simulink model "OMSv1_2"  (Simulink 6.6)
settings: Solver=ode4  SolverMode=SingleTasking  StartTime=0.0  StopTime=5  FixedStep=0.001  MaxStep=0.001  RelTol=1e-3  AbsTol=1e-3
undefined symbols (not defined in the file): alexlaw, bs_onoff, bs_scale, bsfsacrit, bsfsvcrit, cnsgain, fs_onoff, fs_scale, fsdelaycalc, ltdrk, phasicgain, pmcgain, pmctau2, pmctau3, saccsw, spgain, tonicgain, tvrD, tvrN
(part 1 of 7)
CloseFcn:
  | ;slview('closediagram',bdroot);
settings Model: Creator=jacobs  LastModifiedBy=lfd  ExtModeAutoUpdateStatusClock=off
settings DataIOCC: LimitDataPoints=off  SaveOutput=off  SaveTime=off
settings OptimizationCC: BlockReduction=off  BooleanDataType=off
settings DebuggingCC: SignalResolutionControl=TryResolveAllWithWarning  SolverPrmCheckMsg=none  MultiTaskDSMMsg=warning  MultiTaskCondExecSysMsg=none  StrictBusMsg=None
settings HardwareCC: TargetUnknown=on
settings RTWCC: IncludeERTFirstTime=on
settings GRTTargetCC: ModelReferenceCompliant=off  MatFileLogging=off

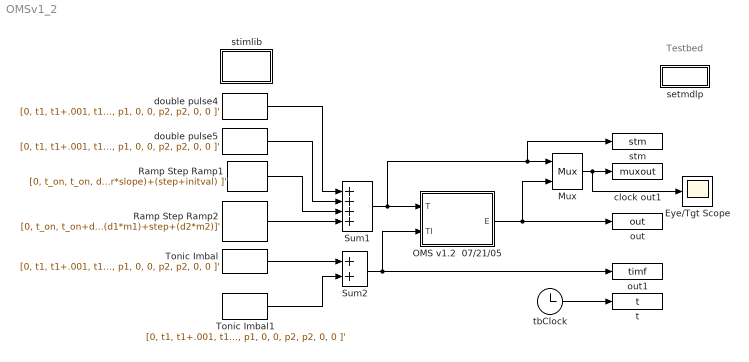
== system OMSv1_2 ==
  note: Testbed
  Eye/Tgt Scope : Scope
      settings: TickLabels=on  TimeRange=5  YMin=-5  YMax=32.5  DataFormat=Array
  Mux : Mux  Inputs=2
  OMS v1.2  07/21/05 : Subsystem
      mask init:
      | k=0.25;loadmdlp;prolong_buffersize=5120;
      mask Display: disp('OMS v1.2\nModel')
  Ramp Step Ramp1 : FromWorkspace  VariableName=[0, t_on, t_on, dur+t_on dur+t_on; initval, initval, initval+step, (dur*slope)+(step+initval), (dur*slope)+(step+initval) ]'  SampleTime=.001  mask{initval=0, t_on=1, step=0, dur=5, slope=0}
      mask prompts: initval "Initial value"; t_on "Time of step"; step "Size of step"; dur "Ramp duration"; slope "Ramp slope"
      mask help: Ramp Step Ramp
      mask Display: disp('Step\nRamp')
  Ramp Step Ramp2 : FromWorkspace  VariableName=[0, t_on, t_on+d1, t_on+d1, t_on+d1+d2, 10000; vi, vi, vi+(d1*m1), (vi+step)+(d1*m1), (vi+step)+(d1*m1)+(d2*m2), vi+(d1*m1)+step+(d2*m2)]'  SampleTime=.001  mask{vi=0, t_on=.25, d1=4, m1=0, step=0, d2=2, m2=0}
      mask prompts: vi "Initial value"; t_on "Time of first ramp"; d1 "First Ramp duration"; m1 "First Ramp slope"; step "Size of step"; d2 "Second Ramp duration"; m2 "Second Ramp slope"
      mask help: Ramp Step Ramp
      mask Display: disp('Ramp\nStep\nRamp')
  Sum1 : Sum  Inputs=++++  SaturateOnIntegerOverflow=on  InputSameDT=on
  Sum2 : Sum  SaturateOnIntegerOverflow=on  InputSameDT=on
  Tonic Imbal : FromWorkspace  VariableName=[0, t1, t1+.001, t1+d1, t1+d1+.001, t1+d1+.001+ipd, t1+d1+.001+ipd, t1+d1+.001+ipd+d2, t1+d1+.001+ipd+d2, 10000; 0, 0, p1, p1, 0, 0, p2, p2, 0, 0 ]'  SampleTime=.001  mask{@1=0, @2=0, @3=2, @4=0, @5=0, @6=3}
      mask prompts: @1 "Pulse 1 Magnitude"; @2 "Time of Pulse 1 Onset"; @3 "Pulse 1 Duration"; @4 "Interpulse Delay"; @5 "Pulse 2 Magnitude"; @6 "Pulse 2 Duration"
      mask help: Double Pulse
      mask init:
      | p1=@1; t1=@2; d1=@3; ipd=@4; p2=@5; d2=@6;
      mask Display: disp('Double\nPulse')
  Tonic Imbal1 : FromWorkspace  VariableName=[0, t1, t1+.001, t1+d1, t1+d1+.001, t1+d1+.001+ipd, t1+d1+.001+ipd, t1+d1+.001+ipd+d2, t1+d1+.001+ipd+d2, 10000; 0, 0, p1, p1, 0, 0, p2, p2, 0, 0 ]'  SampleTime=.001  mask{@1=0, @2=0, @3=3.5, @4=0, @5=0, @6=1.5}
      mask prompts: @1 "Pulse 1 Magnitude"; @2 "Time of Pulse 1 Onset"; @3 "Pulse 1 Duration"; @4 "Interpulse Delay"; @5 "Pulse 2 Magnitude"; @6 "Pulse 2 Duration"
      mask help: Double Pulse
      mask init:
      | p1=@1; t1=@2; d1=@3; ipd=@4; p2=@5; d2=@6;
      mask Display: disp('Double\nPulse')
  clock out1 : ToWorkspace  VariableName=muxout  SaveFormat=Array
      settings: MaxDataPoints=100000
  double pulse4 : FromWorkspace  VariableName=[0, t1, t1+.001, t1+d1, t1+d1+.001, t1+d1+.001+ipd, t1+d1+.001+ipd, t1+d1+.001+ipd+d2, t1+d1+.001+ipd+d2, 10000; 0, 0, p1, p1, 0, 0, p2, p2, 0, 0 ]'  SampleTime=.001  mask{@1=15, @2=2, @3=2, @4=0, @5=0, @6=5}
      mask prompts: @1 "Pulse 1 Magnitude"; @2 "Time of Pulse 1 Onset"; @3 "Pulse 1 Duration"; @4 "Interpulse Delay"; @5 "Pulse 2 Magnitude"; @6 "Pulse 2 Duration"
      mask help: Double Pulse
      mask init:
      | p1=@1; t1=@2; d1=@3; ipd=@4; p2=@5; d2=@6;
      mask Display: disp('Double\nPulse')
  double pulse5 : FromWorkspace  VariableName=[0, t1, t1+.001, t1+d1, t1+d1+.001, t1+d1+.001+ipd, t1+d1+.001+ipd, t1+d1+.001+ipd+d2, t1+d1+.001+ipd+d2, 10000; 0, 0, p1, p1, 0, 0, p2, p2, 0, 0 ]'  SampleTime=.001  mask{@1=0, @2=0, @3=1, @4=0, @5=0, @6=4.5}
      mask prompts: @1 "Pulse 1 Magnitude"; @2 "Time of Pulse 1 Onset"; @3 "Pulse 1 Duration"; @4 "Interpulse Delay"; @5 "Pulse 2 Magnitude"; @6 "Pulse 2 Duration"
      mask help: Double Pulse
      mask init:
      | p1=@1; t1=@2; d1=@3; ipd=@4; p2=@5; d2=@6;
      mask Display: disp('Double\nPulse')
  out : ToWorkspace  VariableName=out  SaveFormat=Array
      settings: MaxDataPoints=100000
  out1 : ToWorkspace  VariableName=timf  SaveFormat=Array
      settings: MaxDataPoints=100000
  setmdlp : Subsystem
      settings: OpenFcn=setmdlp
      mask Display: disp('setmdlp')
  stimlib : Subsystem
      settings: OpenFcn=stimlib
      mask Display: disp('Stimlib')
  stm : ToWorkspace  VariableName=stm  SaveFormat=Array
      settings: MaxDataPoints=100000
  t : ToWorkspace  VariableName=t  SaveFormat=Array
      mask init:
      | global t
      settings: MaxDataPoints=100000
  tbClock : Clock
      settings: Decimation=10
  wires:
  tbClock/1 -> t/1
  double pulse4/1 -> Sum1/1
  Sum1/1 -> OMS v1.2  07/21/05/1(T), stm/1, Mux/1
  OMS v1.2  07/21/05/1(E) -> out/1, Mux/2
  Mux/1 -> clock out1/1, Eye/Tgt Scope/1
  Tonic Imbal/1 -> Sum2/1
  Tonic Imbal1/1 -> Sum2/2
  Sum2/1 -> OMS v1.2  07/21/05/2(TI), out1/1
  double pulse5/1 -> Sum1/2
  Ramp Step Ramp1/1 -> Sum1/3
  Ramp Step Ramp2/1 -> Sum1/4

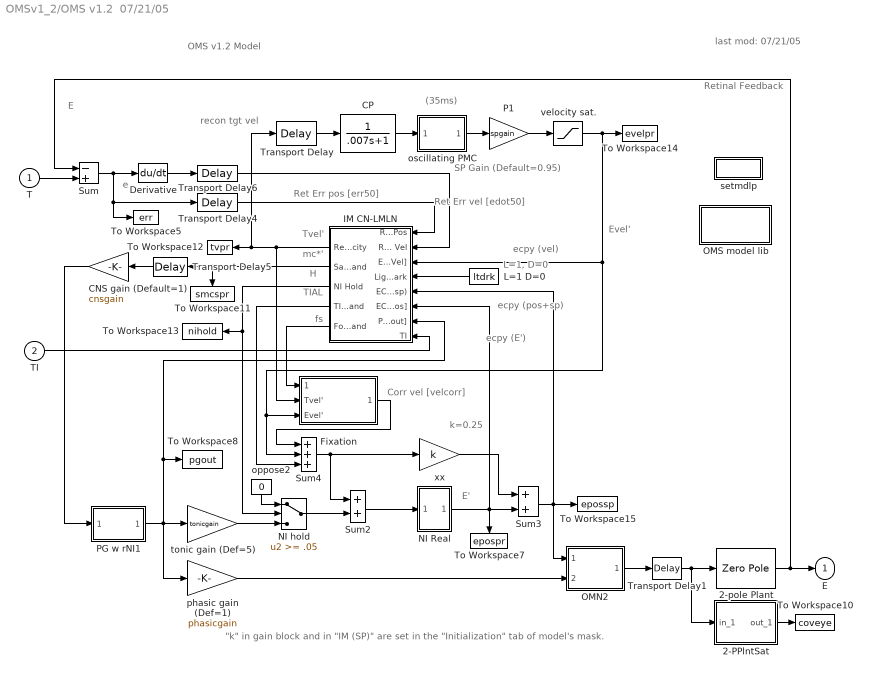
== system OMSv1_2/OMS v1.2  07/21/05 ==
  note: E'
  note: k=0.25
  note: "k" in gain block and in "IM (SP)" are set in
      | the "Initialization" tab of model's mask.
  note: E
  note: e
  note: TIAL
  note: H
  note: mc*'
  note: Tvel'
  note: ecpy
      | (E')
  note: ecpy (vel)
  note: (35ms)
  note: Retinal Feedback
  note: recon tgt vel
  note: last mod:
      | 07/21/05
  note: Evel'
  note: OMS v1.2 Model
  note: ecpy
      | (pos+sp)
  note: Ret Err vel
      | [edot50]
  note: Ret Err pos [err50]
  note: SP Gain
      | (Default=0.95)
  note: L=1, D=0
  note: Corr vel
      | [velcorr]
  note: fs
  T : Inport
  TI : Inport  Port=2
  2-PPlntSat : Subsystem
      mask Display: disp('2-P Plant\n[Sat]')
  2-pole Plant : ZeroPole  Zeros=[ ]  Poles=[ -1/.18 -1/.007]  Gain=[1/.18 * 1/.007]
      mask Display: disp('2-pole\nPlant')
  CNS gain (Default=1) : Gain  Orientation=left  Gain=cnsgain  SaturateOnIntegerOverflow=on
  CP : TransferFcn  Denominator=[.007 1]
  Derivative : Derivative
      mask Display: disp('s')
  Fixation : Subsystem
      mask Display: disp('Fixation')
  IM CN-LMLN : Subsystem  Orientation=left
      mask Display: disp('INTERNAL\nMONITOR')
  L=1 D=0 : Constant  Orientation=left  Value=ltdrk
  NI Real : Subsystem
      mask Display: disp('NI\nReal')
  NI hold : Switch  Threshold=.05  SaturateOnIntegerOverflow=on  InputSameDT=on
  OMN2 : Subsystem
      mask Display: disp('<--"tonic" \nOMN2\n<--"phasic"')
  OMS model lib : Subsystem
      mask Display: disp('OMS Model\nLib')
  P1 : Gain  Gain=spgain  SaturateOnIntegerOverflow=on
  PG w rNI1 : Subsystem
      mask Display: disp('PG rNI\n(2P)')
  Sum : Sum  Inputs=-+  SaturateOnIntegerOverflow=on  InputSameDT=on
  Sum2 : Sum  SaturateOnIntegerOverflow=on  InputSameDT=on
  Sum3 : Sum  SaturateOnIntegerOverflow=on  InputSameDT=on
  Sum4 : Sum  Inputs=+++  SaturateOnIntegerOverflow=on  InputSameDT=on
  To Workspace10 : ToWorkspace  VariableName=coveye  SaveFormat=Array
      settings: MaxDataPoints=10000
  To Workspace11 : ToWorkspace  VariableName=smcspr  SaveFormat=Array
      settings: Orientation=down  MaxDataPoints=10000
  To Workspace12 : ToWorkspace  VariableName=tvpr  SaveFormat=Array
      settings: MaxDataPoints=10000
  To Workspace13 : ToWorkspace  VariableName=nihold  SaveFormat=Array
      settings: MaxDataPoints=10000
  To Workspace14 : ToWorkspace  VariableName=evelpr  SaveFormat=Array
      settings: MaxDataPoints=10000
  To Workspace15 : ToWorkspace  VariableName=epossp  SaveFormat=Array
      settings: MaxDataPoints=10000
  To Workspace5 : ToWorkspace  VariableName=err  SaveFormat=Array
      settings: MaxDataPoints=10000
  To Workspace7 : ToWorkspace  VariableName=epospr  SaveFormat=Array
      settings: Orientation=down  MaxDataPoints=10000
  To Workspace8 : ToWorkspace  VariableName=pgout  SaveFormat=Array
      settings: MaxDataPoints=10000
  Transport Delay : TransportDelay  DelayTime=0.015
      mask Display: disp('15ms')
  Transport Delay1 : TransportDelay  DelayTime=0.03
      mask Display: disp('30ms')
  Transport Delay4 : TransportDelay  DelayTime=.05
      mask Display: disp('50ms')
  Transport Delay5 : TransportDelay  Orientation=left  DelayTime=0.001
      mask Display: disp('1ms')
  Transport Delay6 : TransportDelay  DelayTime=.05
      mask Display: disp('50ms')
  oppose2 : Constant  Orientation=down  Value=0
  oscillating PMC : Subsystem
      mask Display: disp('PMC+')
  phasic gain (Def=1) : Gain  Gain=phasicgain  SaturateOnIntegerOverflow=on
  setmdlp : Subsystem
      settings: OpenFcn=setmdlp
      mask Display: disp('setmdlp')
  tonic gain (Def=5) : Gain  Gain=tonicgain  SaturateOnIntegerOverflow=on
  velocity sat. : Saturate  UpperLimit=90  LowerLimit=-90
  xx : Gain  Gain=k  SaturateOnIntegerOverflow=on
  E : Outport  InitialOutput=0
  wires:
  Derivative/1 -> Transport Delay6/1
  Sum/1 -> Derivative/1, Transport Delay4/1, To Workspace5/1
  T/1 -> Sum/2
  Transport Delay4/1 -> IM CN-LMLN/1(RetErr Pos)
  L=1 D=0/1 -> IM CN-LMLN/4(Light /Dark)
  Transport Delay6/1 -> IM CN-LMLN/2(RetErr Vel)
  CP/1 -> oscillating PMC/1(desired eye vel)
  oscillating PMC/1(efference copy eye vel) -> P1/1
  Transport Delay/1 -> CP/1
  velocity sat./1 -> To Workspace14/1, IM CN-LMLN/3(ECPY [Vel]), Fixation/3(Evel'), Sum4/2
  P1/1 -> velocity sat./1
  TI/1 -> IM CN-LMLN/8(TI)
  IM CN-LMLN/1(Reconstructed Target Velocity) -> To Workspace12/1, Transport Delay/1, Fixation/2(Tvel')
  Sum4/1 -> xx/1, Sum2/1
  IM CN-LMLN/4(TIAL Motor Command) -> Sum4/3
  PG w rNI1/1(PG [pgout]) -> IM CN-LMLN/7(PG [pgout]), To Workspace8/1, tonic gain (Def=5)/1, phasic gain (Def=1)/1
  2-pole Plant/1 -> E/1, Sum/1
  2-PPlntSat/1(out_1) -> To Workspace10/1
  Transport Delay1/1 -> 2-pole Plant/1, 2-PPlntSat/1(in_1)
  tonic gain (Def=5)/1 -> NI hold/3
  phasic gain (Def=1)/1 -> OMN2/2("[pgout]")
  xx/1 -> Sum3/1
  NI Real/1(NIOUT [epospr]) -> Sum3/2, To Workspace7/1, IM CN-LMLN/6(ECPY [Pos])
  Sum3/1 -> IM CN-LMLN/5(ECPY (epossp)), To Workspace15/1, OMN2/1("[epossp]")
  Fixation/1(" CorrVel [velcorr]") -> Sum4/1
  IM CN-LMLN/5(Foveating Saccade Motor  Command) -> Fixation/1(fs [fsmc30])
  oppose2/1 -> NI hold/1
  IM CN-LMLN/3(NI Hold) -> To Workspace13/1, NI hold/2
  IM CN-LMLN/2(Saccadic Motor Command) -> To Workspace11/1, Transport Delay5/1
  Transport Delay5/1 -> CNS gain (Default=1)/1
  CNS gain (Default=1)/1 -> PG w rNI1/1("[mcsprd]")
  Sum2/1 -> NI Real/1(PG + (TIAL+SP))
  NI hold/1 -> Sum2/2
  OMN2/1("[psout]") -> Transport Delay1/1

== system OMSv1_2/setmdlp ==

== system OMSv1_2/stimlib ==

== system OMSv1_2/OMS v1.2  07/21/05/2-PPlntSat ==
  note: A 2-pole plant can be simulated by:
      | 1. no limitation on lateral gaze
      | 2. a hard limitation - placing a saturation in the plant [eg, 55 deg]
      | 3. a soft limitation - add the dead zone  [DZ slope>0]
  in_1 : Inport
  2 pole : ZeroPole  Zeros=[ ]  Poles=[ -1/.18 -1/.007]  Gain=[1/.18 * 1/.007]
      mask Display: disp('2-pole\nPlant')
  DZ slope : Constant  Value=0.05
  Dead Zone : DeadZone  LowerValue=-55  UpperValue=55  SaturateOnIntegerOverflow=on
  Product : Product  SaturateOnIntegerOverflow=on  RndMeth=Zero  InputSameDT=on
  Saturation : Saturate  UpperLimit=55  LowerLimit=-55
  Sum3 : Sum  SaturateOnIntegerOverflow=on  InputSameDT=on
  out_1 : Outport  InitialOutput=0
  wires:
  DZ slope/1 -> Product/2
  Product/1 -> Sum3/2
  Sum3/1 -> out_1/1
  Saturation/1 -> Sum3/1
  Dead Zone/1 -> Product/1
  2 pole/1 -> Saturation/1, Dead Zone/1
  in_1/1 -> 2 pole/1

== system OMSv1_2/OMS v1.2  07/21/05/Fixation ==
  note: Fixation (counter-signal)
  note: Last mod: 02/22/01
  note: Positional error is passed through a gaussian-like function whose greatest
      | response occurs between +/-0.5 deg (approx), corresponding to the sensitivity
      | of the fovea.
  note: This factor is used (with an additional gain factor) to scale the velocity error,
      | which is then subtracted from the velocity signal that is sent from the
      | common neural integrator to the ocular motor neurons.
  note: This should have the effect of reducing the high velocity error (due
      | to CN oscillation or other sources) enough to permit an extension of
      | the foveation period.
  fs [fsmc30] : Inport
  Tvel' : Inport  Port=2
  Evel' : Inport  Port=3
  "30 " : Subsystem  mask{prolong=30}
      mask prompts: prolong "Prolong pulse by?  (msec)"
      mask Display: disp('prolong')
  Boolify2 : Subsystem
      mask Display: disp('Boolify')
  Product : Product  Inputs=3  SaturateOnIntegerOverflow=on  RndMeth=Zero  InputSameDT=on
  Product1 : Product  SaturateOnIntegerOverflow=on  RndMeth=Zero  InputSameDT=on
  Sum5 : Sum  Inputs=+-  SaturateOnIntegerOverflow=on  InputSameDT=on
  Transport Delay7 : TransportDelay  DelayTime=0.050
      mask Display: disp('50ms')
  Vel Sens Factor : Gain  Gain=4  SaturateOnIntegerOverflow=on
  WF % to be applied : Gain  SaturateOnIntegerOverflow=on
  on/off : Constant  Orientation=down
  plantlib link6 : Subsystem
      settings: OpenFcn=fixlib
      mask Display: disp('Fix\nLib')
  velocity sensitivity N : Lookup  InputValues="[-20 -16  -12   -6  -4  4   6   12  16 20]"  OutputValues="[0 0   0.1    0.3    1   1   0.3  0.1   0 0]"  SaturateOnIntegerOverflow=on
  " CorrVel [velcorr]" : Outport  InitialOutput=0
  wires:
  Sum5/1 -> WF % to be applied/1, velocity sensitivity N/1
  Evel'/1 -> Sum5/2
  Tvel'/1 -> Transport Delay7/1
  Transport Delay7/1 -> Sum5/1
  WF % to be applied/1 -> Product/3
  Product1/1 -> " CorrVel [velcorr]"/1
  on/off/1 -> Product1/1
  fs [fsmc30]/1 -> Boolify2/1(In1)
  Boolify2/1(Out1) -> "30 "/1(value(in))
  Vel Sens Factor/1 -> Product/2
  velocity sensitivity N/1 -> Vel Sens Factor/1
  Product/1 -> Product1/2
  "30 "/1(value(out)) -> Product/1

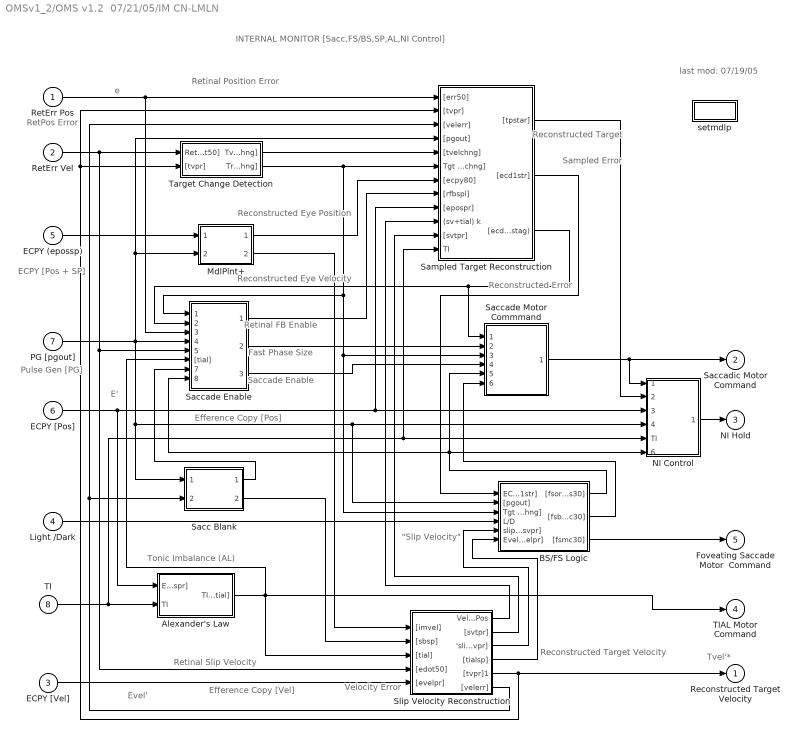
== system OMSv1_2/OMS v1.2  07/21/05/IM CN-LMLN ==
  note: INTERNAL MONITOR [Sacc,FS/BS,SP,AL,NI Control]
  note: last mod:
      | 07/19/05
  note: Reconstructed
      | Target
  note: Sampled
      | Error
  note: Reconstructed
      | Error
  note: Tonic Imbalance (AL)
  note: e
  note: Retinal Position Error
  note: RetPos
      | Error
  note: Reconstructed
      | Eye Position
  note: Reconstructed
      | Eye Velocity
  note: Retinal FB
      | Enable
  note: Saccade
      | Enable
  note: Fast Phase
      | Size
  note: ECPY
      | [Pos
      | + SP]
  note: Pulse
      | Gen
      | [PG]
  note: Evel'
  note: Velocity Error
  note: Retinal Slip Velocity
  note: Efference Copy [Vel]
  note: Reconstructed
      | Target Velocity
  note: Tvel'*
  note: Efference Copy [Pos]
  note: E'
  note: "Slip Velocity"
  RetErr Pos : Inport
  RetErr Vel : Inport  Port=2
  ECPY [Vel] : Inport  Port=3
  Light /Dark : Inport  Port=4
  ECPY (epossp) : Inport  Port=5
  ECPY [Pos] : Inport  Port=6
  PG [pgout] : Inport  Port=7
  TI : Inport  Port=8
  Alexander's Law : Subsystem
      mask Display: disp('Alexander''s\nLaw')
  BS/FS Logic : Subsystem
      mask Display: disp('Braking/Foveating\nSaccade\nLogic')
  MdlPlnt+ : Subsystem
      mask Display: disp('Model\nPlant+')
  NI Control : Subsystem
      mask Display: disp('NI\nControl')
  Sacc Blank : Subsystem
      mask Display: disp('Saccade\n& Drift\nBlanking')
  Saccade Enable : Subsystem
      mask Display: disp('Saccade\nEnable')
  Saccade Motor Commmand : Subsystem
      mask Display: disp('Saccade\nMotor\nCommand')
  Sampled Target Reconstruction : Subsystem
      mask Display: disp('Sampled\nTarget & Error\nReconstruction')
  Slip Velocity Reconstruction : Subsystem
      mask Display: disp('Target &\nSlip Velocity\nReconstruction')
  Target Change Detection : Subsystem
      mask Display: disp('Target Change\nDetection')
  setmdlp : Subsystem
      settings: OpenFcn=setmdlp
      mask Display: disp('setmdlp')
  Reconstructed Target Velocity : Outport  InitialOutput=0
  Saccadic Motor Command : Outport  Port=2  InitialOutput=0
  NI Hold : Outport  Port=3  InitialOutput=0
  TIAL Motor Command : Outport  Port=4  InitialOutput=0
  Foveating Saccade Motor  Command : Outport  Port=5  InitialOutput=0
  wires:
  NI Control/1(Hold [nihold]) -> NI Hold/1
  ECPY [Pos]/1 -> NI Control/3("[epospr]"), Sampled Target Reconstruction/9("[epospr]"), Alexander's Law/1(ECPY [epospr])
  TI/1 -> NI Control/5(TI), Sampled Target Reconstruction/12(TI), Alexander's Law/2(TI)
  PG [pgout]/1 -> Sacc Blank/1(PG [pgout]), NI Control/4(PG [pgout]), BS/FS Logic/2("[pgout]"), Saccade Enable/4("[pgout]"), MdlPlnt+/2("[pgout]"), Sampled Target Reconstruction/4("[pgout]")
  ECPY (epossp)/1 -> MdlPlnt+/1("[epossp]")
  Alexander's Law/1(TIAL [tial]) -> TIAL Motor Command/1, Saccade Enable/6("[tial]"), Slip Velocity Reconstruction/3("[tial]")
  Saccade Motor Commmand/1("[posmc]") -> Saccadic Motor Command/1, NI Control/1("[posmc]")
  Target Change Detection/2(Trgt Chng [tchng]) -> Sampled Target Reconstruction/6(Tgt ch Det [tchng]), Saccade Enable/1(Tgt ch Det [tchng]), BS/FS Logic/3(Tgt ch Det [tchng]), Saccade Motor Commmand/3(Tgt ch Det [tchng])
  RetErr Vel/1 -> Target Change Detection/1(RetErr Vel [edot50]), Saccade Enable/5("[edot50]"), Slip Velocity Reconstruction/4("[edot50]")
  Slip Velocity Reconstruction/1(Vel->Pos) -> Sampled Target Reconstruction/10((sv+tial) k)
  Slip Velocity Reconstruction/2("[svtpr]") -> Sampled Target Reconstruction/11("[svtpr]")
  Slip Velocity Reconstruction/6("[velerr]") -> Sacc Blank/2(RetVelErr [velerr]), Sampled Target Reconstruction/3("[velerr]")
  Target Change Detection/1(Tvel Chng [tvelchng]) -> Sampled Target Reconstruction/5("[tvelchng]")
  Sampled Target Reconstruction/1("[tpstar]") -> NI Control/2(T'* [tpstar])
  RetErr Pos/1 -> Saccade Enable/3("[err50]"), Sampled Target Reconstruction/1("[err50]")
  MdlPlnt+/1("[ecpy80]") -> Sampled Target Reconstruction/7("[ecpy80]")
  Saccade Enable/1("[rfbspl]") -> Sampled Target Reconstruction/8("[rfbspl]")
  Slip Velocity Reconstruction/5("[tvpr]1") -> Target Change Detection/2("[tvpr]"), Sampled Target Reconstruction/2("[tvpr]"), Reconstructed Target Velocity/1
  BS/FS Logic/1("[fsorbs30]") -> NI Control/6("[fsorbs30]"), Saccade Enable/8("[fsorbs30]"), Saccade Motor Commmand/5("[fsorbs30]")
  BS/FS Logic/3("[fsmc30]") -> Foveating Saccade Motor  Command/1
  MdlPlnt+/2("[imvel]") -> Slip Velocity Reconstruction/1("[imvel]")
  Sacc Blank/2(SP S/H [sbsp]) -> Slip Velocity Reconstruction/2("[sbsp]")
  ECPY [Vel]/1 -> Slip Velocity Reconstruction/5("[evelpr]")
  Sampled Target Reconstruction/2("[ecd1str]") -> BS/FS Logic/1(ECD1* [ecd1str])
  Light /Dark/1 -> BS/FS Logic/4(L/D)
  Slip Velocity Reconstruction/3("'slip vel\" [svpr]") -> BS/FS Logic/5(slip vel [svpr])
  Slip Velocity Reconstruction/4("[tialsp]") -> BS/FS Logic/6(Evel' [evelpr])
  Sacc Blank/1(SacBlnk [sbsac]) -> Saccade Enable/7("[sbsac]")
  Sampled Target Reconstruction/3("[ecdstrdz] (excl nystag)") -> Saccade Enable/2("[ecdstrdz]"), Saccade Motor Commmand/1("[ecdstrdz]")
  Saccade Enable/2(FPh Size [fphsz]) -> Saccade Motor Commmand/2("[fphsz]")
  Saccade Enable/3("[sacenab]") -> Saccade Motor Commmand/4("[sacenab]")
  BS/FS Logic/2("[fsbsmc30]") -> Saccade Motor Commmand/6("[fsbcmc30]")

== system OMSv1_2/OMS v1.2  07/21/05/NI Real ==
  note: NI Real
  PG + (TIAL+SP) : Inport
  Gain : Gain  Gain=25  SaturateOnIntegerOverflow=on
  Gain1 : Gain  Orientation=left  SaturateOnIntegerOverflow=on
  Sum : Sum  SaturateOnIntegerOverflow=on  InputSameDT=on
  Transfer Fcn : TransferFcn  Numerator=[1/25]  Denominator=[1 1/25]
  NIOUT [epospr] : Outport  InitialOutput=0
  wires:
  PG + (TIAL+SP)/1 -> Gain/1
  Gain/1 -> Sum/2
  Sum/1 -> Transfer Fcn/1
  Gain1/1 -> Sum/1
  Transfer Fcn/1 -> Gain1/1, NIOUT [epospr]/1

== system OMSv1_2/OMS v1.2  07/21/05/OMN2 ==
  note: OMN
  note: Note that the OMN properly combines the pulse with the output of the NI, by latching
      | that output to its value at the moment the pulse appears.
  note: Operation: when the pulse is active ("from PG") it activates the switch, passing the
      | upper input through to the output.  When the pulse is over, the switch changes,
      | allowing the lower input (from the NI) to pass.
  note: This block behaves like the ocular motor neurons,combining a phasic pulse (from PG)
      | with the tonic step produced by integration of the step, yielding a Pulse-Step
      | to drive the plant.
  "[epossp]" : Inport
  "[pgout]" : Inport  Port=2
  Abs : Abs  SaturateOnIntegerOverflow=on
  Gain _ : Gain  Gain=1.0  SaturateOnIntegerOverflow=on
  SampHold? : Subsystem
      mask Display: disp('H=H\nS=L')
  Sign : Subsystem
      mask Type: Sign
      mask Description: y = sign(x)
      mask Help: Sign Function:\n\t\t\ty = 1 if x > 0\n\t\t\ty = 0 if x = 0\n\t\t\ty = -1 if x < 0
      mask Display: plot(-50,-50,50,50,[-50,50],[0,0],[0,0],[-50,50],[-40,0],[-30,-30],[0,40],[30,30])
  Sum : Sum  SaturateOnIntegerOverflow=on  InputSameDT=on
  Switch : Switch  Threshold=.5  SaturateOnIntegerOverflow=on  InputSameDT=on
  "[psout]" : Outport  InitialOutput=0
  wires:
  "[epossp]"/1 -> Switch/3, SampHold?/1(Input)
  Sign/1(out_1) -> Switch/2, SampHold?/2(S/H?)
  Gain _/1 -> Sum/1
  SampHold?/1(output) -> Sum/2
  Sum/1 -> Switch/1
  "[pgout]"/1 -> Abs/1, Gain _/1
  Switch/1 -> "[psout]"/1
  Abs/1 -> Sign/1(in_1)

== system OMSv1_2/OMS v1.2  07/21/05/OMS model lib ==
  note: How to add your own:
  note: 1. Duplicate on of the existing library blocks above.
  note: 2. In 'Edit' menu, select 'Look under mask'. In 'Icon' tab,
      |    modify the 'disp' statement in the 'Drawing Commands' field
  note: 3. In 'Edit' menu, select "Block Properties', and select the 'Callbacks'
      | tab.  Select 'OpenFcn*' from the Callback function list on the left.
      | Change the content to the name of the library you wish to call.
  plantlib link : Subsystem
      settings: OpenFcn=plantlib
      mask Display: disp('Plant\nLib')
  plantlib link1 : Subsystem
      settings: OpenFcn=nilib
      mask Display: disp('NI\nLib')
  plantlib link2 : Subsystem
      settings: OpenFcn=imlib
      mask Display: disp('IM\nLib')
  plantlib link3 : Subsystem
      settings: OpenFcn=misclib
      mask Display: disp('Misc.\nLib')
  plantlib link4 : Subsystem
      settings: OpenFcn=cnlib
      mask Display: disp('CN\nLib')
  plantlib link5 : Subsystem
      settings: OpenFcn=lnlib
      mask Display: disp('LN\nLib')
  plantlib link6 : Subsystem
      settings: OpenFcn=fixlib
      mask Display: disp('Fix\nLib')
  plantlib link7 : Subsystem
      settings: OpenFcn=filtlib
      mask Display: disp('Filt\nLib')
  stimlib : Subsystem
      settings: OpenFcn=stimlib
      mask Display: disp('Stimlib')

== system OMSv1_2/OMS v1.2  07/21/05/PG w rNI1 ==
  note: Here it is at last!  A pulse generator based on a resettable integrator (look inside the PW
      | block).  The PW function controls the switch, allowing the output of the PH function to pass
      | for the appropriate duration.
  note: The refractory latch prevents the pulse generator from responding to another stimulus until a
      | physiologically acceptable refractory period has elapsed by controlling the "Sample and Hold" block.
  note: PG with Resettable NI
  note: (Init input:0)
  "[mcsprd]" : Inport
  Constant1 : Constant  Orientation=up  Value=0
  PH funct : MATLABFcn  MATLABFcn=phfn_ss
      mask Display: disp('PH\nfunction')
  PW funct : Subsystem
      mask Display: disp('PW\nfunction')
  RefLatch (Default = 50ms) : Subsystem  Orientation=left  mask{@1=saccrefract}
      mask prompts: @1 "Refractory Period (ms)"
      mask help: Refractory Latch
      mask init:
      | delay=@1;
      mask Display: disp('Refract\nLatch')
  SampHold?1 : Subsystem
      mask Display: disp('S=H\nH=L')
  Switch : Switch  Threshold=0.5  SaturateOnIntegerOverflow=on  InputSameDT=on
  loop breaker : Memory  Orientation=left
  PG [pgout] : Outport  InitialOutput=0
  wires:
  Constant1/1 -> Switch/3
  Switch/1 -> loop breaker/1, PG [pgout]/1
  loop breaker/1 -> RefLatch (Default = 50ms)/1(in_1)
  SampHold?1/1(output) -> PH funct/1, PW funct/1(mcspl)
  "[mcsprd]"/1 -> SampHold?1/1(Input)
  PW funct/1(pgw) -> Switch/2
  PH funct/1 -> Switch/1
  RefLatch (Default = 50ms)/1(out_1) -> SampHold?1/2(S/H?)

== system OMSv1_2/OMS v1.2  07/21/05/oscillating PMC ==
  note: desired
      | eye accel
  note: original parameters:
      | tau3=30ms
      | tau2 = 35ms
      | fb gain = 1.1
  note: Robinson: PMC+ block
  note: motor
      | error
  note: efference
      | copy
  note: "Acceleration saturation" can be seen as a lookup table that
      | provides an acceleration for a given input velocity.  We then
      | use an integrator to convert the acceleration back to a velocity.
  note: From: Robinson DA, Gordon JL and Gordon SE
      | A model of smooth pursuit eye movements
      | Biological Cybernetics 55: 43-57,  1986
  note: By increasing feedback gain,
      | above 1.1 (about 2.2)
      | we can make this block oscillate at
      | a lower tau3 than it would otherwise.
  note: CN = 3.025
      | Norm = 1.1
  note: (Default=30ms, CN=40ms)
  note: (Default=35ms)
  note: CN
      | 825
      | 0
      | .002
      | .050
      | -925
      | .002
  note: Normal
      | 0
      | 0
      | .002
      | .050
      | 0
      | .002
  desired eye vel : Inport
  Sum : Sum  Inputs=-++  SaturateOnIntegerOverflow=on  InputSameDT=on
  Transfer Fcn2 : TransferFcn  Numerator=[pmcgain]  Denominator=[1 0]
  accel saturation : MATLABFcn  MATLABFcn=accsat
      mask Display: plot([-80 -4 4 80],[-120 -40 40 120], [0 0],[-120 120],[-80 80],[0 0])
  double pulse4 : FromWorkspace  VariableName=[0, t1, t1+.001, t1+d1, t1+d1+.001, t1+d1+.001+ipd, t1+d1+.001+ipd, t1+d1+.001+ipd+d2, t1+d1+.001+ipd+d2, 10000; 0, 0, p1, p1, 0, 0, p2, p2, 0, 0 ]'  SampleTime=.001  mask{@1=825, @2=0, @3=.002, @4=.050, @5=-925, @6=.002}
      mask prompts: @1 "Pulse 1 Magnitude"; @2 "Time of Pulse 1 Onset"; @3 "Pulse 1 Duration"; @4 "Interpulse Delay"; @5 "Pulse 2 Magnitude"; @6 "Pulse 2 Duration"
      mask help: Double Pulse
      mask init:
      | p1=@1; t1=@2; d1=@3; ipd=@4; p2=@5; d2=@6;
      mask Display: disp('Double\nPulse')
  tau2 : TransportDelay  DelayTime=pmctau2/1000
  tau3 : TransportDelay  Orientation=left  DelayTime=pmctau3/1000
  efference copy eye vel : Outport  InitialOutput=0
  wires:
  accel saturation/1 -> tau2/1
  tau2/1 -> Transfer Fcn2/1
  Sum/1 -> accel saturation/1
  tau3/1 -> Sum/1
  desired eye vel/1 -> Sum/2
  Transfer Fcn2/1 -> efference copy eye vel/1, tau3/1
  double pulse4/1 -> Sum/3

== system OMSv1_2/OMS v1.2  07/21/05/setmdlp ==

== system OMSv1_2/OMS v1.2  07/21/05/Fixation/30  ==
  note: init = 0
  note: init = 0
  note: 02/16/01
  note: The start of the input pulse causes the value on input 1 to be held starting when the leading
      | edge occurs, and this value remains latched until 'delay' seconds after the pulse ends (trailing edge).
  note: The two integration step delays before the S&H block's S/H (bottom) input insures
      | that the input value to be latched is available to theS&H block's top input
      | before the S&H block tries to 'hold'.
  note: Stretch the duration of an input pulse, latching it at its value at pulse onset.
  note: init Q = 0
  note: Changed from 1 to 2 delays
      | on 2/16/01 to provide insurance that
      | the signal at the S input will be available
  value(in) : Inport
  " x/1000" : Constant  Orientation=up  Value=0.001
  Latch1 : Subsystem  mask(Latch){@1=0}
      mask prompts: @1 "Initial State for Output "Q":"
      mask help: Latch
      mask init:
      | ini=(@1~=0);
      mask Help: Latches the S input.  When S (set) is one, the Q output  becomes one.  The output remains one until the R (reset) input becomes one, forcing the output to zero.  If both R and S are one, the latch will be in an undefined state.
      mask Display: disp('S   Q\n\nR  !Q')
  Product : Product  SaturateOnIntegerOverflow=on  RndMeth=Zero  InputSameDT=on
  SampHold?2 : Subsystem
      mask Display: disp('S=L\nH=H')
  Terminator : Terminator
  Variable Transport Delay : VariableTransportDelay  MaximumDelay=10  MaximumPoints=prolong_buffersize
  leading edge detect : Subsystem
      mask Display: disp('Leading\nEdge Det')
  loop breaker2 : Memory
  loop breaker3 : Memory
  stretch : Constant  Value=prolong
  trailing edge detect : Subsystem
      mask Display: disp('Trailing\nEdge Det')
  value(out) : Outport  InitialOutput=0
  wires:
  " x/1000"/1 -> Product/2
  Product/1 -> Variable Transport Delay/2
  stretch/1 -> Product/1
  SampHold?2/1(output) -> value(out)/1
  trailing edge detect/1(out_1) -> Variable Transport Delay/1
  value(in)/1 -> SampHold?2/1(Input), trailing edge detect/1(in_1), leading edge detect/1(in_1)
  Latch1/1(out_1) -> loop breaker2/1
  loop breaker2/1 -> loop breaker3/1
  loop breaker3/1 -> SampHold?2/2(S/H?)
  leading edge detect/1(out_1) -> Latch1/1(in_1)
  Variable Transport Delay/1 -> Latch1/2(in_2)
  Latch1/2(out_2) -> Terminator/1

== system OMSv1_2/OMS v1.2  07/21/05/Fixation/Boolify2 ==
  In1 : Inport
  Abs2 : Abs  SaturateOnIntegerOverflow=on
  direction1 : Subsystem
      mask Type: Sign
      mask Description: y = sign(x)
      mask Help: Sign Function:\n\t\t\ty = 1 if x > 0\n\t\t\ty = 0 if x = 0\n\t\t\ty = -1 if x < 0
      mask Display: plot(-50,-50,50,50,[-50,50],[0,0],[0,0],[-50,50],[-40,0],[-30,-30],[0,40],[30,30])
  Out1 : Outport  InitialOutput=0
  wires:
  Abs2/1 -> direction1/1(in_1)
  In1/1 -> Abs2/1
  direction1/1(out_1) -> Out1/1

== system OMSv1_2/OMS v1.2  07/21/05/Fixation/plantlib link6 ==

== system OMSv1_2/OMS v1.2  07/21/05/IM CN-LMLN/Alexander's Law ==
  note: Alexander's law
  ECPY [epospr] : Inport
  TI : Inport  Port=2
  'alexlaw' (via 'setmdlp') : Gain  Gain=alexlaw  SaturateOnIntegerOverflow=on
  Boolify : Subsystem
      mask Display: disp('Boolify')
  Product : Product  SaturateOnIntegerOverflow=on  RndMeth=Zero  InputSameDT=on
  Product1 : Product  SaturateOnIntegerOverflow=on  RndMeth=Zero  InputSameDT=on
  Relational Operator : RelationalOperator  InputSameDT=on
  Relational Operator1 : RelationalOperator  Operator=<=  InputSameDT=on
  Sum : Sum  SaturateOnIntegerOverflow=on  InputSameDT=on
  Switch5 : Switch  SaturateOnIntegerOverflow=on  InputSameDT=on
  Switch6 : Switch  Threshold=.25  SaturateOnIntegerOverflow=on  InputSameDT=on
  Transfer Fcn : TransferFcn  Numerator=[5]  Denominator=[1 5]
  direction : Subsystem
      mask Type: Sign
      mask Description: y = sign(x)
      mask Help: Sign Function:\n\t\t\ty = 1 if x > 0\n\t\t\ty = 0 if x = 0\n\t\t\ty = -1 if x < 0
      mask Display: plot(-50,-50,50,50,[-50,50],[0,0],[0,0],[-50,50],[-40,0],[-30,-30],[0,40],[30,30])
  oppose1 : Constant  Orientation=up  Value=0
  oppose2 : Constant  Orientation=up  Value=0
  TIAL [tial] : Outport  InitialOutput=0
  wires:
  ECPY [epospr]/1 -> 'alexlaw' (via 'setmdlp')/1
  'alexlaw' (via 'setmdlp')/1 -> Transfer Fcn/1
  Transfer Fcn/1 -> Sum/1
  Sum/1 -> Product1/1, Relational Operator1/1, Product/2, Relational Operator/1
  Relational Operator/1 -> Product1/2
  Product1/1 -> Switch5/1
  Relational Operator1/1 -> Product/1
  Product/1 -> Switch5/3
  oppose1/1 -> Relational Operator/2, Relational Operator1/2
  TI/1 -> Boolify/1(TI), Sum/2, direction/1(in_1)
  Switch5/1 -> Switch6/1
  Switch6/1 -> TIAL [tial]/1
  oppose2/1 -> Switch6/3
  direction/1(out_1) -> Switch5/2
  Boolify/1(Switch Control) -> Switch6/2

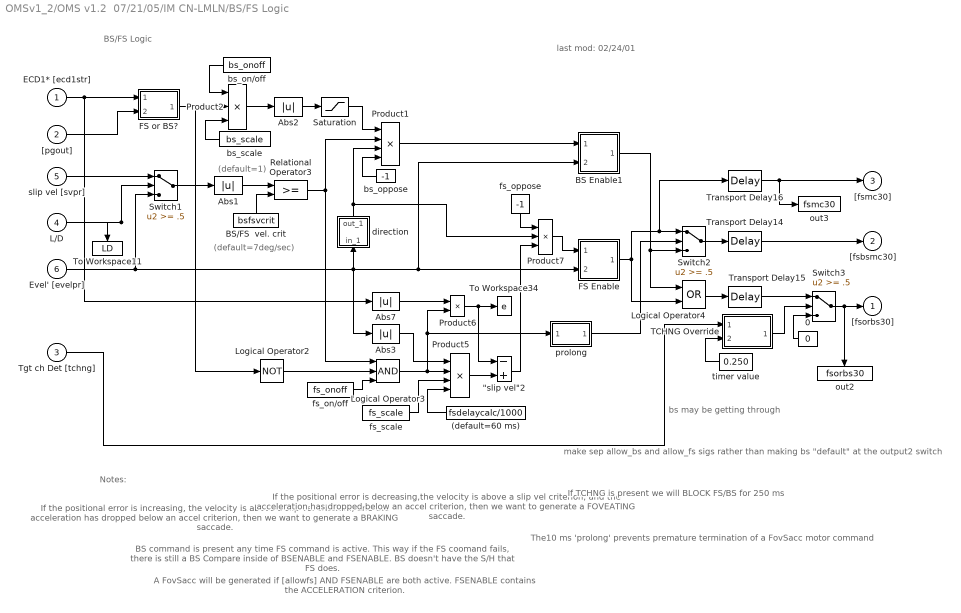
== system OMSv1_2/OMS v1.2  07/21/05/IM CN-LMLN/BS/FS Logic ==
  note: BS/FS Logic
  note: If the positional error is increasing, the velocity
      |  is above a slip vel criterion, and the acceleration
      | has dropped below an accel criterion, then we
      | want to generate a BRAKING saccade.
  note: If the positional error is decreasing,the velocity
      | is above a slip vel criterion, and the acceleration
      | has dropped below an accel criterion, then we
      | want to generate a FOVEATING saccade.
  note: last mod:
      | 02/24/01
  note: (default=7deg/sec)
  note: (default=1)
  note: If TCHNG is present we will BLOCK
      | FS/BS for 250 ms
  note: BS command is present any time FS command is active.  This way if the FS coomand fails, there is still a BS
      | Compare inside of BSENABLE and FSENABLE.  BS doesn't have the S/H that FS does.
  note: A FovSacc will be generated if [allowfs] AND FSENABLE are both active. FSENABLE contains the ACCELERATION criterion.
  note: Notes:
  note: The10 ms 'prolong' prevents premature
      | termination of a FovSacc motor command
  note: make sep allow_bs and allow_fs
      | sigs rather than making bs "default"
      | at the output2 switch
  note: bs may be getting through
  ECD1* [ecd1str] : Inport
  "[pgout]" : Inport  Port=2
  Tgt ch Det [tchng] : Inport  Port=3
  L/D : Inport  Port=4
  slip vel [svpr] : Inport  Port=5
  Evel' [evelpr] : Inport  Port=6
  "\"slip vel\"2" : Sum  Inputs=-+  SaturateOnIntegerOverflow=on  InputSameDT=on
  (default=60 ms) : Constant  Orientation=left  Value=fsdelaycalc/1000
  0 : Constant  Orientation=left  Value=0
  Abs{1..3,7} (4 alike) : Abs  SaturateOnIntegerOverflow=on
  BS Enable1 : Subsystem
      mask Display: disp('BS\nEnab')
  BS/FS  vel. crit : Constant  Orientation=up  Value=bsfsvcrit
  FS Enable : Subsystem
      mask Display: disp('FS\nEnab')
  FS or BS? : Subsystem
      mask Display: disp('BS=1\nFS=0')
  Logical Operator2 : Logic  Operator=NOT  Inputs=1
  Logical Operator3 : Logic  Inputs=3
  Logical Operator4 : Logic  Operator=OR
  Product1 : Product  Inputs=4  SaturateOnIntegerOverflow=on  RndMeth=Zero  InputSameDT=on
  Product2 : Product  Inputs=3  SaturateOnIntegerOverflow=on  RndMeth=Zero  InputSameDT=on
  Product5 : Product  Inputs=4  SaturateOnIntegerOverflow=on  RndMeth=Zero  InputSameDT=on
  Product6 : Product  SaturateOnIntegerOverflow=on  RndMeth=Zero  InputSameDT=on
  Product7 : Product  Inputs=3  SaturateOnIntegerOverflow=on  RndMeth=Zero  InputSameDT=on
  Relational Operator3 : RelationalOperator  InputSameDT=on
  Saturation : Saturate  UpperLimit=2  LowerLimit=0
  Switch1 : Switch  Threshold=.5  SaturateOnIntegerOverflow=on  InputSameDT=on
  Switch2 : Switch  Threshold=.5  SaturateOnIntegerOverflow=on  InputSameDT=on
  Switch3 : Switch  Threshold=.5  SaturateOnIntegerOverflow=on  InputSameDT=on
  TCHNG Override : Subsystem
      mask Display: disp('TCHNG\nOverride')
  To Workspace11 : ToWorkspace  VariableName=LD  SaveFormat=Array
      settings: Orientation=down  MaxDataPoints=10000
  To Workspace34 : ToWorkspace  VariableName=e  SaveFormat=Array
      settings: MaxDataPoints=10000
  Transport Delay14 : TransportDelay  DelayTime=0.03
      mask Display: disp('30ms')
  Transport Delay15 : TransportDelay  DelayTime=0.03
      mask Display: disp('30ms')
  Transport Delay16 : TransportDelay  DelayTime=0.03
      mask Display: disp('30ms')
  bs_on/off : Constant  Orientation=left  Value=bs_onoff
  bs_oppose : Constant  Orientation=left  Value=-1
  bs_scale : Constant  Orientation=left  Value=bs_scale
  direction : Subsystem  Orientation=up
      mask Type: Sign
      mask Description: y = sign(x)
      mask Help: Sign Function:\n\t\t\ty = 1 if x > 0\n\t\t\ty = 0 if x = 0\n\t\t\ty = -1 if x < 0
      mask Display: plot(-50,-50,50,50,[-50,50],[0,0],[0,0],[-50,50],[-40,0],[-30,-30],[0,40],[30,30])
  fs_on/off : Constant  Value=fs_onoff
  fs_oppose : Constant  Orientation=down  Value=-1
  fs_scale : Constant  Value=fs_scale
  out2 : ToWorkspace  VariableName=fsorbs30  SaveFormat=Array
      settings: Orientation=down  MaxDataPoints=100000
  out3 : ToWorkspace  VariableName=fsmc30  SaveFormat=Array
      settings: MaxDataPoints=100000
  prolong : Subsystem  mask{prolong=1}
      mask prompts: prolong "Prolong pulse by?  (msec)"
      mask Display: disp('prolong')
  timer value : Constant  Orientation=left  Value=0.250
  "[fsorbs30]" : Outport  InitialOutput=0
  "[fsbsmc30]" : Outport  Port=2  InitialOutput=0
  "[fsmc30]" : Outport  Port=3  InitialOutput=0
  wires:
  Abs2/1 -> Saturation/1
  FS or BS?/1(BS=1 FS=0) -> Product2/2, Logical Operator2/1
  bs_on/off/1 -> Product2/1
  bs_scale/1 -> Product2/3
  slip vel [svpr]/1 -> Switch1/1
  Switch1/1 -> Abs1/1
  Evel' [evelpr]/1 -> Switch1/3, direction/1(in_1), BS Enable1/2("[evelpr]"), FS Enable/2("[evelpr]"), Abs3/1
  Relational Operator3/1 -> Logical Operator3/1, Product1/2
  "[pgout]"/1 -> FS or BS?/2(pgout)
  ECD1* [ecd1str]/1 -> FS or BS?/1(pos error [ecd1str]), Abs7/1
  BS/FS  vel. crit/1 -> Relational Operator3/2
  Abs1/1 -> Relational Operator3/1
  bs_oppose/1 -> Product1/4
  direction/1(out_1) -> Product1/3, Product7/2
  Logical Operator2/1 -> Logical Operator3/2
  (default=60 ms)/1 -> Product5/4
  Abs3/1 -> Product5/1
  Logical Operator3/1 -> Product5/2, Product6/2, prolong/1(value(in))
  fs_oppose/1 -> Product7/1
  Abs7/1 -> Product6/1
  Product6/1 -> "\"slip vel\"2"/1, To Workspace34/1
  FS Enable/1("[fsmc]") -> Switch2/1, Transport Delay16/1, Logical Operator4/2
  Switch2/1 -> Transport Delay14/1
  fs_scale/1 -> Product5/3
  fs_on/off/1 -> Logical Operator3/3
  Tgt ch Det [tchng]/1 -> TCHNG Override/1("[tchng]")
  timer value/1 -> TCHNG Override/2(timer dur)
  Transport Delay14/1 -> "[fsbsmc30]"/1
  Transport Delay15/1 -> Switch3/1
  0/1 -> Switch3/3
  TCHNG Override/1(tchng sw) -> Switch3/2
  Transport Delay16/1 -> "[fsmc30]"/1, out3/1
  Product2/1 -> Abs2/1
  Saturation/1 -> Product1/1
  Product5/1 -> "\"slip vel\"2"/2
  "\"slip vel\"2"/1 -> Product7/3
  Product7/1 -> FS Enable/1(fsprod)
  Product1/1 -> BS Enable1/1(bsprod)
  BS Enable1/1("[bsmc]") -> Switch2/3, Logical Operator4/1
  Logical Operator4/1 -> Transport Delay15/1
  prolong/1(value(out)) -> Switch2/2
  Switch3/1 -> "[fsorbs30]"/1, out2/1
  L/D/1 -> Switch1/2, To Workspace11/1

== system OMSv1_2/OMS v1.2  07/21/05/IM CN-LMLN/MdlPlnt+ ==
  note: Plant Model+
  note: last mod:
      | 01/31/00
  "[epossp]" : Inport
  "[pgout]" : Inport  Port=2
  "\"Plant\"" : ZeroPole  Zeros=[ ]  Poles=[ -1/.18 -1/.007]  Gain=[1/.18 * 1/.007]
      mask Display: disp('2-pole\n"Plant"')
  Derivative : Derivative
      mask Display: disp('s')
  OMN2 : Subsystem
      mask Display: disp('<--tonic\nOMN2\n<--phasic')
  To Workspace13 : ToWorkspace  VariableName=ecpy80  SaveFormat=Array
      settings: MaxDataPoints=10000
  To Workspace28 : ToWorkspace  VariableName=imvel  SaveFormat=Array
      settings: Orientation=down  MaxDataPoints=10000
      mask Type: imsw1in
  Transport Delay11 : TransportDelay  DelayTime=0.030
      mask Display: disp('30ms')
  Transport Delay12 : TransportDelay  DelayTime=0.050
      mask Display: disp('50ms')
  Transport Delay13 : TransportDelay  DelayTime=0.050
      mask Display: disp('50ms')
  "[ecpy80]" : Outport  InitialOutput=0
  "[imvel]" : Outport  Port=2  InitialOutput=0
  wires:
  "[pgout]"/1 -> OMN2/2("[pgout]")
  "[epossp]"/1 -> OMN2/1("[epossp]")
  Derivative/1 -> Transport Delay13/1
  "\"Plant\""/1 -> Transport Delay12/1, Derivative/1
  Transport Delay11/1 -> "\"Plant\""/1
  OMN2/1(out_1) -> Transport Delay11/1
  Transport Delay12/1 -> "[ecpy80]"/1, To Workspace13/1
  Transport Delay13/1 -> "[imvel]"/1, To Workspace28/1

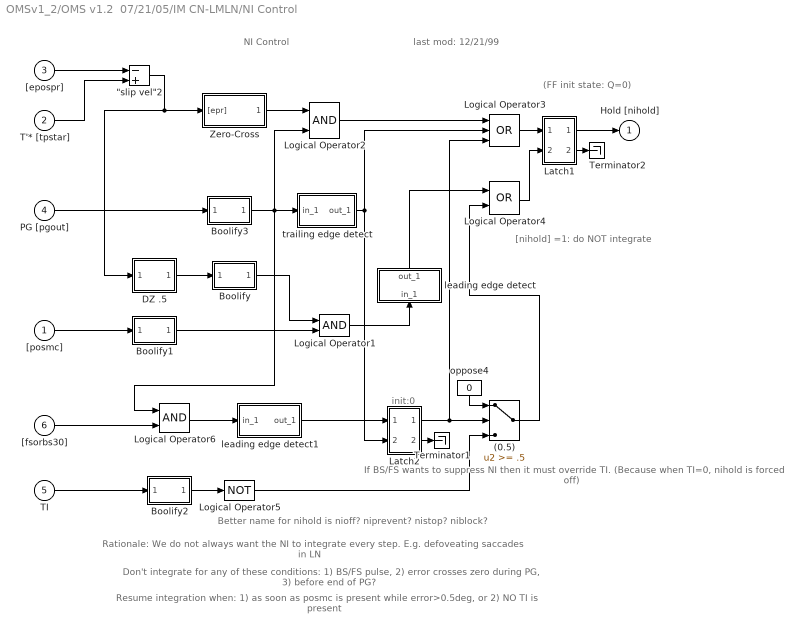
== system OMSv1_2/OMS v1.2  07/21/05/IM CN-LMLN/NI Control ==
  note: (FF init state: Q=0)
  note: NI Control
  note: If BS/FS wants to suppress NI
      | then it must override TI. (Because
      | when TI=0, nihold is forced off)
  note: last mod:
      | 12/21/99
  note: Rationale: We do not always want the NI to integrate every step. E.g. defoveating saccades in LN
  note: Don't integrate for any of these conditions: 1) BS/FS pulse, 2) error crosses zero during PG, 3) before end of PG?
  note: [nihold] =1: do NOT integrate
  note: init:0
  note: Better name for nihold is nioff? niprevent? nistop? niblock?
  note: Resume integration when: 1) as soon as posmc is present while error>0.5deg, or 2) NO TI is present
  "[posmc]" : Inport
  T'* [tpstar] : Inport  Port=2
  "[epospr]" : Inport  Port=3
  PG [pgout] : Inport  Port=4
  TI : Inport  Port=5
  "[fsorbs30]" : Inport  Port=6
  "\"slip vel\"2" : Sum  Inputs=-+  SaturateOnIntegerOverflow=on  InputSameDT=on
  (0.5) : Switch  Threshold=.5  SaturateOnIntegerOverflow=on  InputSameDT=on
  Boolify : Subsystem
      mask Display: disp('Boolify')
  Boolify1 : Subsystem
      mask Display: disp('Boolify')
  Boolify2 : Subsystem
      mask Display: disp('Boolify')
  Boolify3 : Subsystem
      mask Display: disp('Boolify')
  DZ .5 : Subsystem
      mask Display: disp('Dead\nZone')
  Latch1 : Subsystem  mask(Latch){@1=0}
      mask prompts: @1 "Initial State for Output "Q":"
      mask help: Latch
      mask init:
      | ini=(@1~=0);
      mask Help: Latches the S input.  When S (set) is one, the Q output  becomes one.  The output remains one until the R (reset) input becomes one, forcing the output to zero.  If both R and S are one, the latch will be in an undefined state.
      mask Display: disp('S   Q\n\nR  !Q')
  Latch2 : Subsystem  mask(Latch){@1=0}
      mask prompts: @1 "Initial State for Output "Q":"
      mask help: Latch
      mask init:
      | ini=(@1~=0);
      mask Help: Latches the S input.  When S (set) is one, the Q output  becomes one.  The output remains one until the R (reset) input becomes one, forcing the output to zero.  If both R and S are one, the latch will be in an undefined state.
      mask Display: disp('S   Q\n\nR  !Q')
  Logical Operator1 : Logic
  Logical Operator2 : Logic
  Logical Operator3 : Logic  Operator=OR  Inputs=3
  Logical Operator4 : Logic  Operator=OR
  Logical Operator5 : Logic  Operator=NOT  Inputs=1
  Logical Operator6 : Logic
  Terminator1 : Terminator
  Terminator2 : Terminator
  Zero-Cross : Subsystem
      mask Display: disp('Zero-Cross\nDetect')
  leading edge detect : Subsystem  Orientation=up
      mask Display: disp('Leading\nEdge Det')
  leading edge detect1 : Subsystem
      mask Display: disp('Leading\nEdge Det')
  oppose4 : Constant  Orientation=down  Value=0
  trailing edge detect : Subsystem
      mask Display: disp('Trailing\nEdge Det')
  Hold [nihold] : Outport  InitialOutput=0
  wires:
  T'* [tpstar]/1 -> "\"slip vel\"2"/2
  PG [pgout]/1 -> Boolify3/1(In1)
  "[epospr]"/1 -> "\"slip vel\"2"/1
  Latch1/1(out_1) -> Hold [nihold]/1
  Logical Operator1/1 -> leading edge detect/1(in_1)
  "[fsorbs30]"/1 -> Logical Operator6/2
  Latch2/1(out_1) -> Logical Operator3/3, (0.5)/2
  oppose4/1 -> (0.5)/1
  Logical Operator5/1 -> (0.5)/3
  TI/1 -> Boolify2/1(In1)
  Boolify2/1(Out1) -> Logical Operator5/1
  (0.5)/1 -> Logical Operator4/2
  Boolify3/1(Out1) -> Logical Operator6/1, trailing edge detect/1(in_1), Logical Operator2/2
  trailing edge detect/1(out_1) -> Latch2/2(in_2), Logical Operator3/2
  "[posmc]"/1 -> Boolify1/1(In1)
  "\"slip vel\"2"/1 -> DZ .5/1(in_1), Zero-Cross/1("[epr]")
  Zero-Cross/1("[epneq]") -> Logical Operator2/1
  Logical Operator2/1 -> Logical Operator3/1
  Logical Operator3/1 -> Latch1/1(in_1)
  Logical Operator4/1 -> Latch1/2(in_2)
  leading edge detect/1(out_1) -> Logical Operator4/1
  Boolify/1(Out1) -> Logical Operator1/1
  DZ .5/1(out_1) -> Boolify/1(In1)
  Boolify1/1(Out1) -> Logical Operator1/2
  Logical Operator6/1 -> leading edge detect1/1(in_1)
  leading edge detect1/1(out_1) -> Latch2/1(in_1)
  Latch2/2(out_2) -> Terminator1/1
  Latch1/2(out_2) -> Terminator2/1

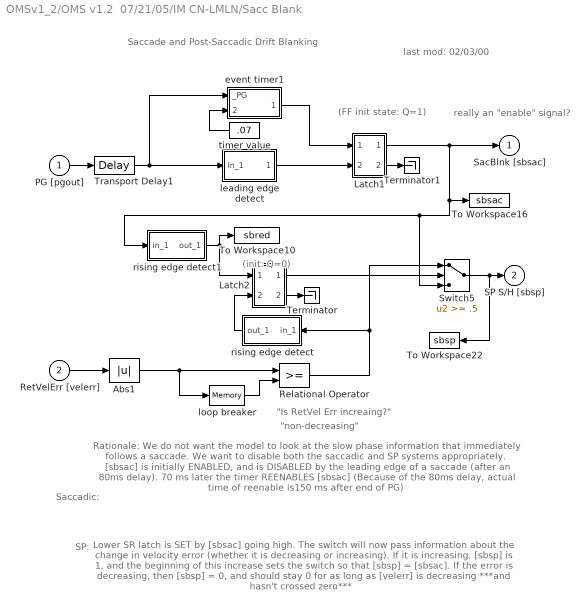
== system OMSv1_2/OMS v1.2  07/21/05/IM CN-LMLN/Sacc Blank ==
  note: Saccade and Post-Saccadic Drift Blanking
  note: (FF init state: Q=1)
  note: "Is RetVel Err increaing?"
  note: really an "enable"
      | signal?
  note: last mod:
      | 02/03/00
  note: [sbsac]  is initially ENABLED, and is DISABLED by  the leading edge of a saccade
      |  (after an 80ms delay).  70 ms later the timer REENABLES [sbsac]
      | (Because of the 80ms delay, actual time of reenable is150 ms after end of PG)
  note: Lower SR latch is SET by [sbsac] going high.  The switch will now pass information
      | about the change in velocity error (whether it is decreasing or increasing).
      | If it is increasing, [sbsp] is 1, and the beginning of this increase sets the switch so
      | that [sbsp] = [sbsac].  If the error is decreasing, then [sbsp] = 0, and should stay 0
      |  for as long as [velerr] is decreasing ***and hasn't crossed zero***
  note: Rationale: We do not want the model to look at the slow phase information that immediately
      | follows a saccade.   We want to disable both the saccadic and SP systems appropriately.
  note: Saccadic:
  note: SP:
  note: (init: Q=0)
  note: "non-decreasing"
  PG [pgout] : Inport
  RetVelErr [velerr] : Inport  Port=2
  Abs1 : Abs  SaturateOnIntegerOverflow=on
  Latch1 : Subsystem  mask(Latch){@1=1}
      mask prompts: @1 "Initial State for Output "Q":"
      mask help: Latch
      mask init:
      | ini=(@1~=0);
      mask Help: Latches the S input.  When S (set) is one, the Q output  becomes one.  The output remains one until the R (reset) input becomes one, forcing the output to zero.  If both R and S are one, the latch will be in an undefined state.
      mask Display: disp('S   Q\n\nR  !Q')
  Latch2 : Subsystem  mask(Latch){@1=0}
      mask prompts: @1 "Initial State for Output "Q":"
      mask help: Latch
      mask init:
      | ini=(@1~=0);
      mask Help: Latches the S input.  When S (set) is one, the Q output  becomes one.  The output remains one until the R (reset) input becomes one, forcing the output to zero.  If both R and S are one, the latch will be in an undefined state.
      mask Display: disp('S   Q\n\nR  !Q')
  Relational Operator : RelationalOperator  InputSameDT=on
  Switch5 : Switch  Threshold=.5  SaturateOnIntegerOverflow=on  InputSameDT=on
  Terminator : Terminator
  Terminator1 : Terminator
  To Workspace10 : ToWorkspace  VariableName=sbred  SaveFormat=Array
      settings: MaxDataPoints=10000
  To Workspace16 : ToWorkspace  VariableName=sbsac  SaveFormat=Array
      settings: MaxDataPoints=10000
  To Workspace22 : ToWorkspace  VariableName=sbsp  SaveFormat=Array
      settings: MaxDataPoints=10000
  Transport Delay1 : TransportDelay  DelayTime=0.080
      mask Display: disp('80ms')
  event timer1 : Subsystem
      mask Display: disp('Event\nTimer2')
  leading edge detect : Subsystem
      mask Display: disp('Leading\nEdge Det')
  loop breaker : Memory
  rising edge detect : Subsystem  Orientation=left
      mask Display: disp('Rising\nEdge Det')
  rising edge detect1 : Subsystem
      mask Display: disp('Rising\nEdge Det')
  timer value : Constant  Orientation=left  Value=.07
  SacBlnk [sbsac] : Outport  InitialOutput=0
  SP S/H [sbsp] : Outport  Port=2  InitialOutput=0
  wires:
  leading edge detect/1(out_1) -> Latch1/2(in_2)
  event timer1/1(out_1) -> Latch1/1(in_1)
  loop breaker/1 -> Relational Operator/2
  Abs1/1 -> loop breaker/1, Relational Operator/1
  Relational Operator/1 -> rising edge detect/1(in_1), Switch5/1
  rising edge detect1/1(out_1) -> To Workspace10/1, Latch2/1(in_1)
  RetVelErr [velerr]/1 -> Abs1/1
  PG [pgout]/1 -> Transport Delay1/1
  Transport Delay1/1 -> leading edge detect/1(in_1), event timer1/1(_PG)
  timer value/1 -> event timer1/2(_timer value (port))
  Latch1/1(out_1) -> SacBlnk [sbsac]/1, rising edge detect1/1(in_1), Switch5/3, To Workspace16/1
  rising edge detect/1(out_1) -> Latch2/2(in_2)
  Latch2/1(out_1) -> Switch5/2
  Switch5/1 -> SP S/H [sbsp]/1, To Workspace22/1
  Latch2/2(out_2) -> Terminator/1
  Latch1/2(out_2) -> Terminator1/1

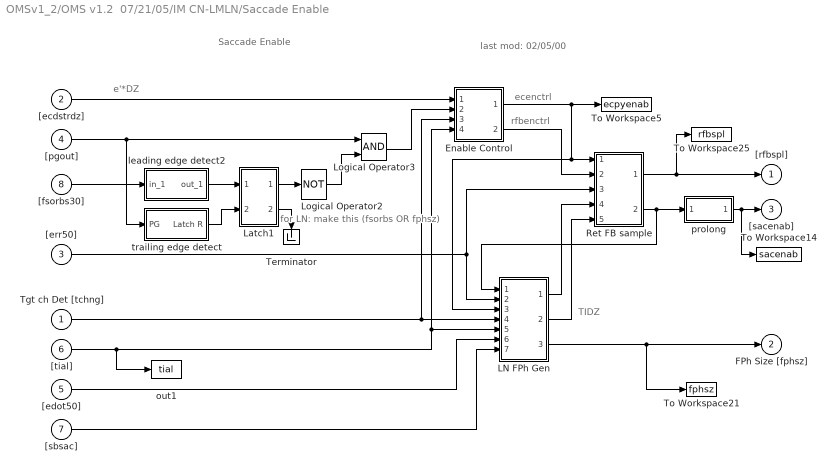
== system OMSv1_2/OMS v1.2  07/21/05/IM CN-LMLN/Saccade Enable ==
  note: Saccade Enable
  note: last mod:
      | 02/05/00
  note: rfbenctrl
  note: ecenctrl
  note: e'*DZ
  note: for LN: make this
      | (fsorbs OR fphsz)
  note: TIDZ
  Tgt ch Det [tchng] : Inport
  "[ecdstrdz]" : Inport  Port=2
  "[err50]" : Inport  Port=3
  "[pgout]" : Inport  Port=4
  "[edot50]" : Inport  Port=5
  "[tial]" : Inport  Port=6
  "[sbsac]" : Inport  Port=7
  "[fsorbs30]" : Inport  Port=8
  Enable Control : Subsystem
      mask Display: disp('Enable\nControl')
  LN FPh Gen : Subsystem
      mask Display: disp('DFFPh\nGen')
  Latch1 : Subsystem  mask(Latch){@1=0}
      mask prompts: @1 "Initial State for Output "Q":"
      mask help: Latch
      mask init:
      | ini=(@1~=0);
      mask Help: Latches the S input.  When S (set) is one, the Q output  becomes one.  The output remains one until the R (reset) input becomes one, forcing the output to zero.  If both R and S are one, the latch will be in an undefined state.
      mask Display: disp('S   Q\n\nR  !Q')
  Logical Operator2 : Logic  Operator=NOT  Inputs=1
  Logical Operator3 : Logic
  Ret FB sample : Subsystem
      mask Display: disp('Ret FB\nEnab &\nSample')
  Terminator : Terminator
      settings: Orientation=down
  To Workspace14 : ToWorkspace  VariableName=sacenab  SaveFormat=Array
      settings: MaxDataPoints=10000
      mask Type: imsw1in
  To Workspace21 : ToWorkspace  VariableName=fphsz  SaveFormat=Array
      settings: MaxDataPoints=10000
  To Workspace25 : ToWorkspace  VariableName=rfbspl  SaveFormat=Array
      settings: MaxDataPoints=10000
      mask Type: imsw1in
  To Workspace5 : ToWorkspace  VariableName=ecpyenab  SaveFormat=Array
      settings: MaxDataPoints=10000
      mask Type: imsw1in
  leading edge detect2 : Subsystem
      mask Display: disp('Leading\nEdge Det')
  out1 : ToWorkspace  VariableName=tial  SaveFormat=Array
      settings: MaxDataPoints=100000
  prolong : Subsystem  mask{prolong=10}
      mask prompts: prolong "Prolong pulse by?  (msec)"
      mask Display: disp('prolong')
  trailing edge detect : Subsystem
      mask Display: disp('Trailing\nEdge Det')
  "[rfbspl]" : Outport  InitialOutput=0
  FPh Size [fphsz] : Outport  Port=2  InitialOutput=0
  "[sacenab]" : Outport  Port=3  InitialOutput=0
  wires:
  "[pgout]"/1 -> Logical Operator3/1, trailing edge detect/1(PG)
  Logical Operator2/1 -> Logical Operator3/2
  "[ecdstrdz]"/1 -> Enable Control/1(e'*DZ [ecdstrdz])
  Tgt ch Det [tchng]/1 -> LN FPh Gen/4(TCD [tchng]), Enable Control/3(Tgt ch Det [tchng])
  "[sbsac]"/1 -> LN FPh Gen/7("[sbsac]")
  "[edot50]"/1 -> LN FPh Gen/6("[edot50]")
  Enable Control/1(ECPY EnTmng [ecpyenab]) -> LN FPh Gen/3("[ecpyenab]"), Ret FB sample/1("[ecpyenab]"), To Workspace5/1
  "[err50]"/1 -> LN FPh Gen/2("[err50]"), Ret FB sample/3("[err50]")
  Enable Control/2(RetFB En&Spl) -> Ret FB sample/2("[rfbenctrl]")
  LN FPh Gen/2(TIDZ) -> Ret FB sample/5(TIDZ)
  Ret FB sample/2(RetFB Enable [sacenab]) -> prolong/1(value(in)), LN FPh Gen/1("[rfbenab]")
  "[fsorbs30]"/1 -> leading edge detect2/1(in_1)
  leading edge detect2/1(out_1) -> Latch1/1(in_1)
  Latch1/1(out_1) -> Logical Operator2/1
  trailing edge detect/1(Latch R) -> Latch1/2(in_2)
  Logical Operator3/1 -> Enable Control/2(VolPG ( [pgout] &NOT fs or bs))
  LN FPh Gen/1("[eedot]") -> Ret FB sample/4("[eedot]")
  Ret FB sample/1(RFB Spl [rfbspl]) -> "[rfbspl]"/1, To Workspace25/1
  LN FPh Gen/3(FPh Size [fphsz]) -> FPh Size [fphsz]/1, To Workspace21/1
  prolong/1(value(out)) -> "[sacenab]"/1, To Workspace14/1
  "[tial]"/1 -> LN FPh Gen/5("[tial]"), Enable Control/4("[tial]"), out1/1
  Latch1/2(out_2) -> Terminator/1
